simulink model "V126_L1_UMS"  (R2020b)
settings: Solver=VariableStepAuto  StartTime=0.0  StopTime=600  MaxStep=0.01  RelTol=1e-3
undefined symbols (not defined in the file): Kp
settings Model: Creator=td  LastModifiedBy=Maxim
settings DataIOCC: ReturnWorkspaceOutputs=off
settings DebuggingCC: ArithmeticOperatorsInVariantConditions=warning
settings SFSimCC: CustomCodeUndefinedFunction=UseInterfaceOnly

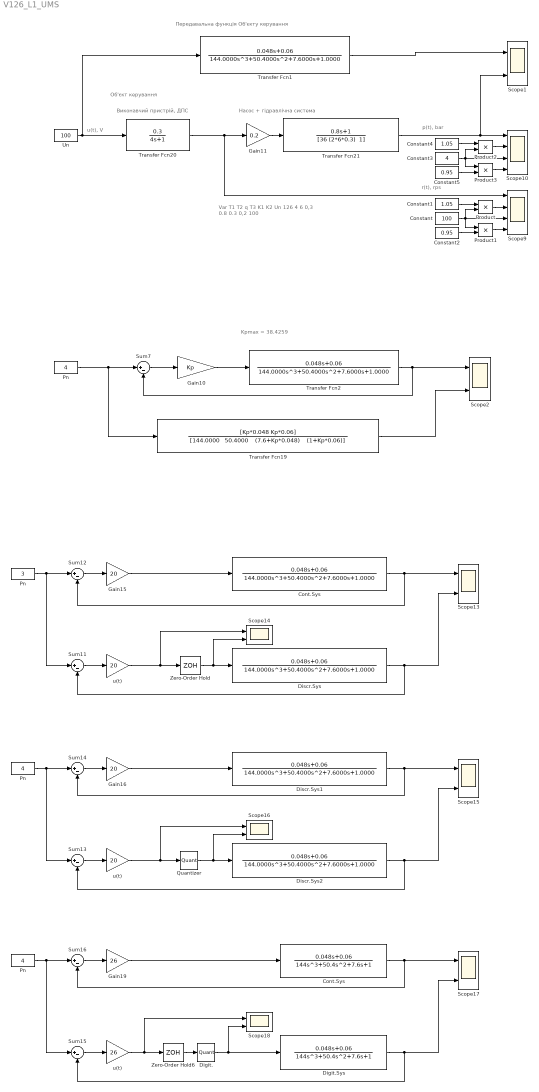
== system V126_L1_UMS ==
  note: Передавальна функція Об'єкту керування
  note: Kpmax = 38.4259
  note: Var	T1	T2	q	T3	K1	K2	Un
      | 126	4	6	0,3	0.8	0.3	0,2	100
  note: p(t), bar
  note: u(t), V
  note: Насос + гідравлічна система
  note: r(t), rps
  note: Виконавчий пристрій, ДПС
  note: Об'єкт керування
  " Pn" : Constant  Value=4
  " Pn " : Constant  Value=4
  " Quantizer " : Quantizer  QuantizationInterval=0.1
  " Zero-Order Hold " : ZeroOrderHold  SampleTime=0.01
  " u(t)   " : Gain  Gain=26
  Constant : Constant  Value=100
  Constant1 : Constant  Value=1.05
  Constant2 : Constant  Value=0.95
  Constant3 : Constant  Value=4
  Constant4 : Constant  Value=1.05
  Constant5 : Constant  Value=0.95
  Cont.Sys : TransferFcn  Numerator=[0.048 0.06]  Denominator="[144.0000   50.4000    7.6000    1.0000]"
  "Cont.Sys    " : TransferFcn  Numerator=[0.048 0.06]  Denominator=[144 50.4 7.6 1]
  Digit. : Quantizer
  "Digit.Sys  " : TransferFcn  Numerator=[0.048 0.06]  Denominator=[144 50.4 7.6 1]
  Discr.Sys : TransferFcn  Numerator=[0.048 0.06]  Denominator="[144.0000   50.4000    7.6000    1.0000]"
  Discr.Sys1 : TransferFcn  Numerator=[0.048 0.06]  Denominator="[144.0000   50.4000    7.6000    1.0000]"
  Discr.Sys2 : TransferFcn  Numerator=[0.048 0.06]  Denominator="[144.0000   50.4000    7.6000    1.0000]"
  Gain10 : Gain  Gain=Kp
  Gain11 : Gain  Gain=0.2
  Gain15 : Gain  Gain=20
  Gain16 : Gain  Gain=20
  Gain19 : Gain  Gain=26
  Pn : Constant  Value=4
  "Pn " : Constant  Value=3
  Product{,1..3} (4 alike) : Product
  Scope{1..2,13..18} (8 alike) : Scope  NumInputPorts=2
  Scope10 : Scope  NumInputPorts=4
  Scope9 : Scope  NumInputPorts=4
  Sum{7,11..16} (7 alike) : Sum  Inputs=|+-
  Transfer Fcn1 : TransferFcn  Numerator=[0.048 0.06]  Denominator="[144.0000   50.4000    7.6000    1.0000]"
  Transfer Fcn19 : TransferFcn  Numerator=[Kp*0.048 Kp*0.06]  Denominator="[144.0000   50.4000    (7.6+Kp*0.048)    (1+Kp*0.06)]"
  Transfer Fcn2 : TransferFcn  Numerator=[0.048 0.06]  Denominator="[144.0000   50.4000    7.6000    1.0000]"
  Transfer Fcn20 : TransferFcn  Numerator=[0.3]  Denominator=[4 1]
  Transfer Fcn21 : TransferFcn  Numerator=[0.8 1]  Denominator="[36 (2*6*0.3)  1]"
  Un : Constant  Value=100
  Zero-Order Hold6 : ZeroOrderHold  SampleTime=0.02
  u(t) : Gain  Gain=20
  "u(t) " : Gain  Gain=20
  wires:
  Un/1 -> Transfer Fcn1/1, Transfer Fcn20/1
  Constant5/1 -> Product3/2
  Product1/1 -> Scope9/4
  Product3/1 -> Scope10/4
  Transfer Fcn20/1 -> Scope9/1, Gain11/1
  Constant4/1 -> Product2/1
  Constant3/1 -> Product2/2, Product3/1, Scope10/3
  Product2/1 -> Scope10/2
  Gain11/1 -> Transfer Fcn21/1
  Transfer Fcn21/1 -> Scope1/2, Scope10/1
  Product/1 -> Scope9/2
  Constant2/1 -> Product1/2
  Constant/1 -> Product/2, Product1/1, Scope9/3
  Constant1/1 -> Product/1
  Transfer Fcn1/1 -> Scope1/1
  Gain10/1 -> Transfer Fcn2/1
  Pn/1 -> Transfer Fcn19/1, Sum7/1
  Transfer Fcn2/1 -> Sum7/2, Scope2/1
  Transfer Fcn19/1 -> Scope2/2
  Sum7/1 -> Gain10/1
  Sum13/1 -> "u(t) "/1
  "Pn "/1 -> Sum11/1, Sum12/1
  " Quantizer "/1 -> Discr.Sys2/1, Scope16/2
  Discr.Sys1/1 -> Scope15/1, Sum14/2
  Sum15/1 -> " u(t)   "/1
  Gain19/1 -> "Cont.Sys    "/1
  "Digit.Sys  "/1 -> Scope17/2, Sum15/2
  " Pn "/1 -> Sum15/1, Sum16/1
  Digit./1 -> "Digit.Sys  "/1, Scope18/2
  u(t)/1 -> Scope14/1, " Zero-Order Hold "/1
  Sum16/1 -> Gain19/1
  Gain15/1 -> Cont.Sys/1
  " Pn"/1 -> Sum13/1, Sum14/1
  " Zero-Order Hold "/1 -> Discr.Sys/1, Scope14/2
  Zero-Order Hold6/1 -> Digit./1
  Gain16/1 -> Discr.Sys1/1
  Cont.Sys/1 -> Scope13/1, Sum12/2
  "Cont.Sys    "/1 -> Scope17/1, Sum16/2
  " u(t)   "/1 -> Zero-Order Hold6/1, Scope18/1
  Sum12/1 -> Gain15/1
  "u(t) "/1 -> " Quantizer "/1, Scope16/1
  Discr.Sys2/1 -> Scope15/2, Sum13/2
  Sum11/1 -> u(t)/1
  Sum14/1 -> Gain16/1
  Discr.Sys/1 -> Scope13/2, Sum11/2
